simulink model "Dual_Sliding_Surface_Control_Try2"  (R2021b)
settings: Solver=VariableStepAuto  StartTime=tspan(1)  StopTime=tspan(2)  MinStep=1e-4  RelTol=1e-7
undefined symbols (not defined in the file): lambda_beta_num, lambda_gamma_num, lambda_x_num, lambda_y_num, r_sim, x_0
libraries: simulink_extras x2
settings Model: Creator=domin  LastModifiedBy=domin
settings SolverCC: AlgebraicLoopSolver=TrustRegion
settings DebuggingCC: SFMachineParentedDataDiag=warning

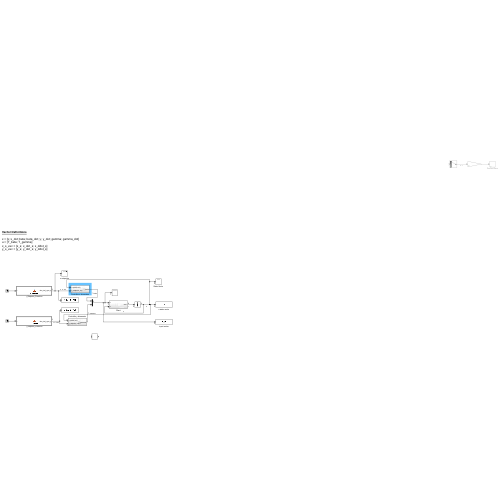
[thumbnail: Simulink's stored preview of the top-level diagram]
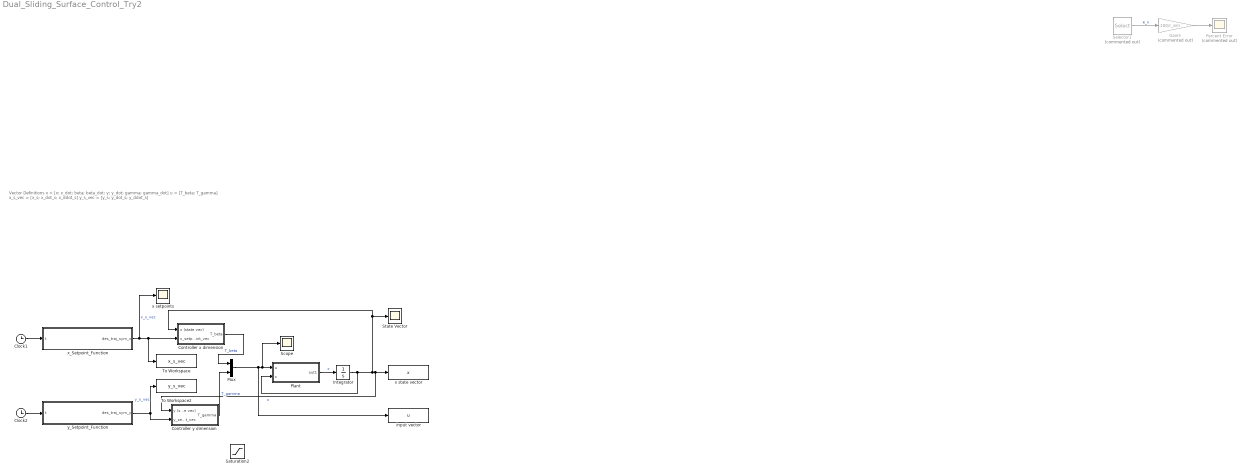
== system Dual_Sliding_Surface_Control_Try2 ==
  note: Vector Definitions
      |
      | x = [x; x_dot; beta; beta_dot; y; y_dot; gamma; gamma_dot]
      | u = [T_beta; T_gamma]
      | x_s_vec = [x_s; x_dot_s; x_ddot_s]
      | y_s_vec = [y_s; y_dot_s; y_ddot_s]
  Clock1 : Clock
  Clock2 : Clock
  Controller x dimension : Subsystem
  Controller y dimension : Subsystem
  Gain5 : Gain  Commented=on  Gain=100/r_sim
  Integrator : Integrator  InitialCondition=x_0
  Mux : Mux  Inputs=2
  Percent Error : Scope  Commented=on
  Plant : Subsystem
  Saturation2 : Saturate  UpperLimit=75/1000  LowerLimit=-75/1000  ZeroCross=off
  Scope : Scope
  Selector1 : Selector  Commented=on  InputPortWidth=5  IndexOptions=Index vector (dialog)  Indices=[1]  OutputSizes=1
  State Vector : Scope
  To Workspace : ToWorkspace  VariableName=x_s_vec  SampleTime=-1
  To Workspace2 : ToWorkspace  VariableName=y_s_vec  SampleTime=-1
  input vector : ToWorkspace  VariableName=u  SampleTime=-1
  x setpoints : Scope
  x state vector : ToWorkspace  VariableName=x  SampleTime=-1
  x_Setpoint_Function : MATLAB Function  TreatAsAtomicUnit=on
  y_Setpoint_Function : MATLAB Function  TreatAsAtomicUnit=on
  wires:
  x_Setpoint_Function/1(des_traj_sym_x) -> x setpoints/1, To Workspace/1, Controller x dimension/2(x_setpoint_vec)  "x_s_vec"
  Integrator/1 -> Plant/2(x), Controller y dimension/1(y (state vec)), x state vector/1, Controller x dimension/1(x (state vec)), State Vector/1  "x"
  Plant/1(out1) -> Integrator/1  "x"
  Clock1/1 -> x_Setpoint_Function/1(t)
  Gain5/1 -> Percent Error/1
  Selector1/1 -> Gain5/1  "e_x"
  Clock2/1 -> y_Setpoint_Function/1(t)
  Controller x dimension/1(T_beta) -> Mux/1  "T_beta"
  Controller y dimension/1(T_gamma) -> Mux/2  "T_gamma"
  y_Setpoint_Function/1(des_traj_sym_y) -> Controller y dimension/2(y_setpoint_vec), To Workspace2/1  "y_s_vec"
  Mux/1 -> Scope/1, Plant/1(u), input vector/1

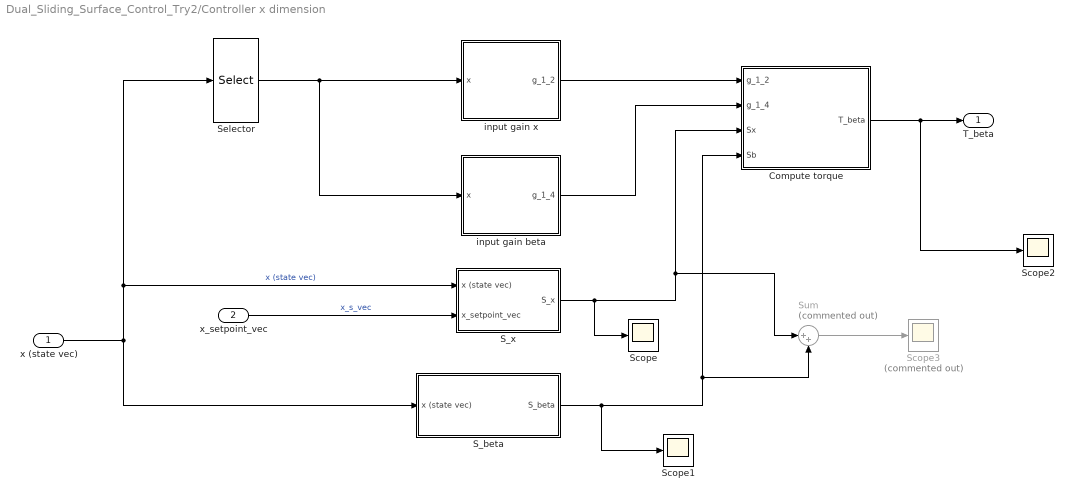
== system Dual_Sliding_Surface_Control_Try2/Controller x dimension ==
  x (state vec) : Inport
  x_setpoint_vec : Inport  Port=2
  Compute torque : MATLAB Function  TreatAsAtomicUnit=on
  S_beta : Subsystem
  S_x : Subsystem
  Scope : Scope
  Scope1 : Scope
  Scope2 : Scope
  Scope3 : Scope  Commented=on
  Selector : Selector  InputPortWidth=8  IndexOptions=Index vector (dialog)  Indices=[1]  OutputSizes=1
  Sum : Sum  Commented=on  Inputs=|++
  input gain beta : MATLAB Function  TreatAsAtomicUnit=on
  input gain x : MATLAB Function  TreatAsAtomicUnit=on
  T_beta : Outport
  wires:
  x (state vec)/1 -> Selector/1, S_x/1(x (state vec)), S_beta/1(x (state vec))  "x (state vec)"
  Selector/1 -> input gain beta/1(x), input gain x/1(x)
  x_setpoint_vec/1 -> S_x/2(x_setpoint_vec)  "x_s_vec"
  input gain x/1(g_1_2) -> Compute torque/1(g_1_2)
  input gain beta/1(g_1_4) -> Compute torque/2(g_1_4)
  S_x/1(S_x) -> Scope/1, Sum/1, Compute torque/3(Sx)
  S_beta/1(S_beta) -> Scope1/1, Sum/2, Compute torque/4(Sb)
  Compute torque/1(T_beta) -> T_beta/1, Scope2/1
  Sum/1 -> Scope3/1

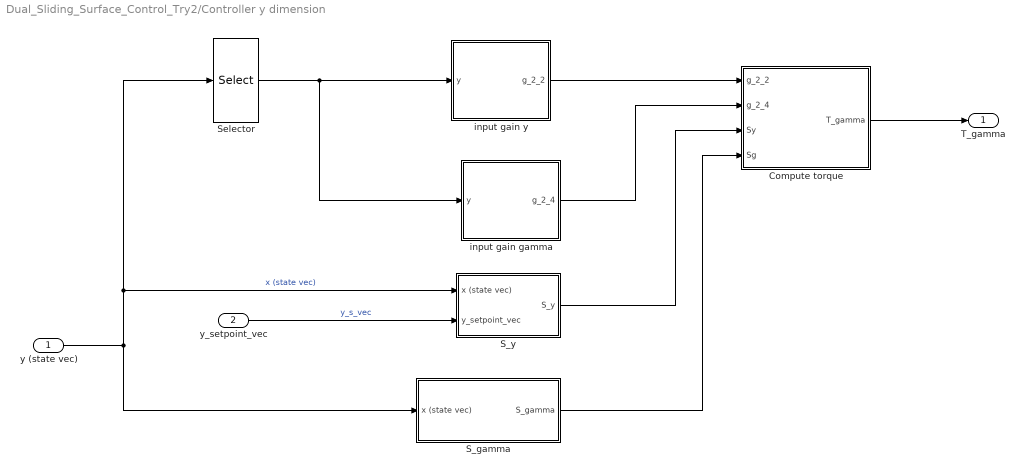
== system Dual_Sliding_Surface_Control_Try2/Controller y dimension ==
  y (state vec) : Inport
  y_setpoint_vec : Inport  Port=2
  Compute torque : MATLAB Function  TreatAsAtomicUnit=on
  S_gamma : Subsystem
  S_y : Subsystem
  Selector : Selector  InputPortWidth=8  IndexOptions=Index vector (dialog)  Indices=[5]  OutputSizes=1
  input gain gamma : MATLAB Function  TreatAsAtomicUnit=on
  input gain y : MATLAB Function  TreatAsAtomicUnit=on
  T_gamma : Outport
  wires:
  S_y/1(S_y) -> Compute torque/3(Sy)
  Compute torque/1(T_gamma) -> T_gamma/1
  input gain y/1(g_2_2) -> Compute torque/1(g_2_2)
  Selector/1 -> input gain gamma/1(y), input gain y/1(y)
  y_setpoint_vec/1 -> S_y/2(y_setpoint_vec)  "y_s_vec"
  input gain gamma/1(g_2_4) -> Compute torque/2(g_2_4)
  y (state vec)/1 -> Selector/1, S_y/1(x (state vec)), S_gamma/1(x (state vec))  "x (state vec)"
  S_gamma/1(S_gamma) -> Compute torque/4(Sg)

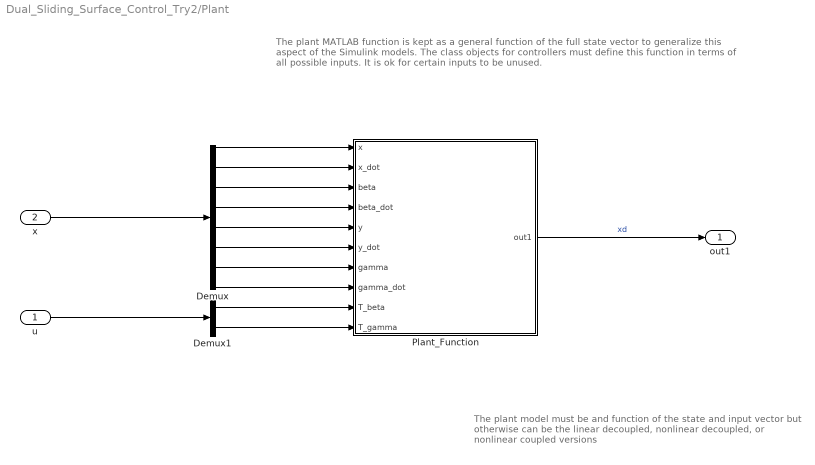
== system Dual_Sliding_Surface_Control_Try2/Plant ==
  note: The plant MATLAB function is kept as a general function of the full state vector
      | to generalize this aspect of the Simulink models. The class objects for controllers must define this function in terms of all possible inputs. It is ok for certain inputs to be unused.
  note: The plant model must be and function of the state and input vector
      |  but otherwise can be the linear decoupled, nonlinear decoupled,
      | or nonlinear coupled versions
  u : Inport
  x : Inport  Port=2
  Demux : Demux  Outputs=8
  Demux1 : Demux  Outputs=2
  Plant_Function : MATLAB Function  TreatAsAtomicUnit=on
  out1 : Outport
  wires:
  Demux1/1 -> Plant_Function/9(T_beta)
  Demux1/2 -> Plant_Function/10(T_gamma)
  Demux/5 -> Plant_Function/5(y)
  Demux/8 -> Plant_Function/8(gamma_dot)
  Demux/7 -> Plant_Function/7(gamma)
  Demux/1 -> Plant_Function/1(x)
  Demux/3 -> Plant_Function/3(beta)
  Demux/4 -> Plant_Function/4(beta_dot)
  Demux/2 -> Plant_Function/2(x_dot)
  Demux/6 -> Plant_Function/6(y_dot)
  x/1 -> Demux/1
  Plant_Function/1(out1) -> out1/1  "xd"
  u/1 -> Demux1/1

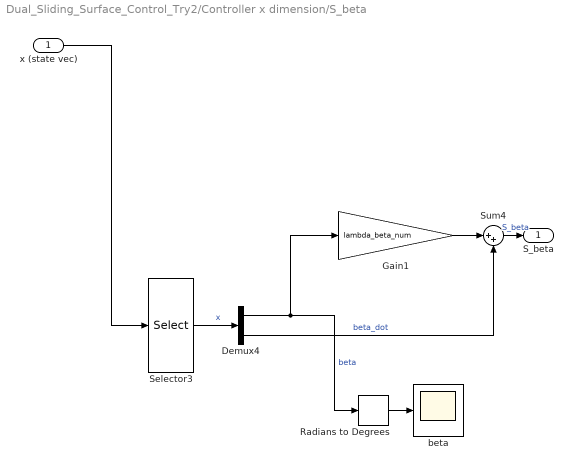
== system Dual_Sliding_Surface_Control_Try2/Controller x dimension/S_beta ==
  x (state vec) : Inport
  Demux4 : Demux  Outputs=2
  Gain1 : Gain  Gain=lambda_beta_num
  Radians to Degrees : simulink_extras/Transformations/Radians to Degrees
  Selector3 : Selector  InputPortWidth=8  IndexOptions=Index vector (dialog)  Indices=[3 4]  OutputSizes=1
  Sum4 : Sum  Inputs=|++
  beta : Scope
  S_beta : Outport
  wires:
  x (state vec)/1 -> Selector3/1
  Sum4/1 -> S_beta/1  "S_beta"
  Demux4/1 -> Gain1/1, Radians to Degrees/1  "beta"
  Gain1/1 -> Sum4/1
  Demux4/2 -> Sum4/2  "beta_dot"
  Radians to Degrees/1 -> beta/1
  Selector3/1 -> Demux4/1  "x"

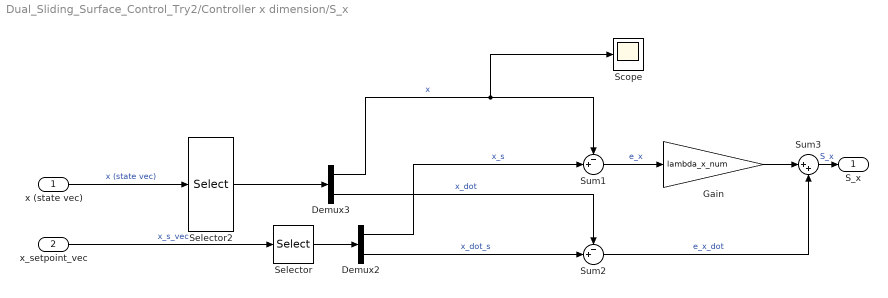
== system Dual_Sliding_Surface_Control_Try2/Controller x dimension/S_x ==
  x (state vec) : Inport
  x_setpoint_vec : Inport  Port=2
  Demux2 : Demux  Outputs=2
  Demux3 : Demux  Outputs=2
  Gain : Gain  Gain=lambda_x_num
  Scope : Scope
  Selector : Selector  InputPortWidth=3  IndexOptions=Index vector (dialog)  Indices=[1 2]  OutputSizes=1
  Selector2 : Selector  InputPortWidth=8  IndexOptions=Index vector (dialog)  Indices=[1 2]  OutputSizes=1
  Sum1 : Sum  Inputs=-+|
  Sum2 : Sum  Inputs=-+|
  Sum3 : Sum  Inputs=|++
  S_x : Outport
  wires:
  Gain/1 -> Sum3/1
  Sum1/1 -> Gain/1  "e_x"
  Sum2/1 -> Sum3/2  "e_x_dot"
  Demux3/1 -> Scope/1, Sum1/1  "x"
  Demux3/2 -> Sum2/1  "x_dot"
  Sum3/1 -> S_x/1  "S_x"
  x_setpoint_vec/1 -> Selector/1  "x_s_vec"
  x (state vec)/1 -> Selector2/1  "x (state vec)"
  Demux2/2 -> Sum2/2  "x_dot_s"
  Demux2/1 -> Sum1/2  "x_s"
  Selector2/1 -> Demux3/1
  Selector/1 -> Demux2/1

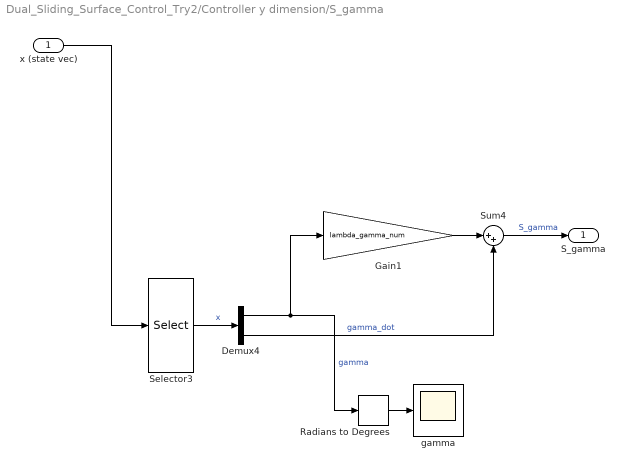
== system Dual_Sliding_Surface_Control_Try2/Controller y dimension/S_gamma ==
  x (state vec) : Inport
  Demux4 : Demux  Outputs=2
  Gain1 : Gain  Gain=lambda_gamma_num
  Radians to Degrees : simulink_extras/Transformations/Radians to Degrees
  Selector3 : Selector  InputPortWidth=8  IndexOptions=Index vector (dialog)  Indices=[7 8]  OutputSizes=1
  Sum4 : Sum  Inputs=|++
  gamma : Scope
  S_gamma : Outport
  wires:
  x (state vec)/1 -> Selector3/1
  Sum4/1 -> S_gamma/1  "S_gamma"
  Demux4/1 -> Gain1/1, Radians to Degrees/1  "gamma"
  Gain1/1 -> Sum4/1
  Demux4/2 -> Sum4/2  "gamma_dot"
  Radians to Degrees/1 -> gamma/1
  Selector3/1 -> Demux4/1  "x"

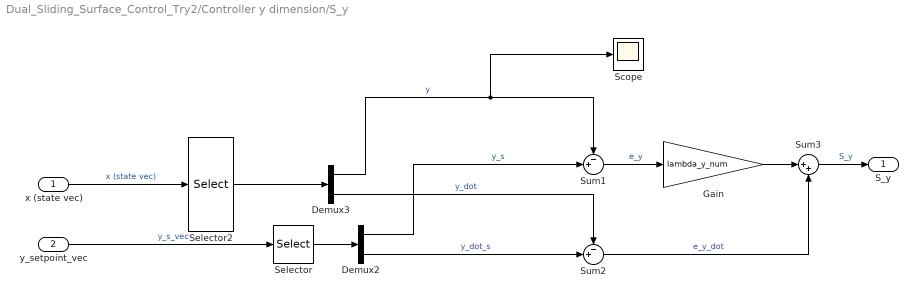
== system Dual_Sliding_Surface_Control_Try2/Controller y dimension/S_y ==
  x (state vec) : Inport
  y_setpoint_vec : Inport  Port=2
  Demux2 : Demux  Outputs=2
  Demux3 : Demux  Outputs=2
  Gain : Gain  Gain=lambda_y_num
  Scope : Scope
  Selector : Selector  InputPortWidth=3  IndexOptions=Index vector (dialog)  Indices=[1 2]  OutputSizes=1
  Selector2 : Selector  InputPortWidth=8  IndexOptions=Index vector (dialog)  Indices=[5 6]  OutputSizes=1
  Sum1 : Sum  Inputs=-+|
  Sum2 : Sum  Inputs=-+|
  Sum3 : Sum  Inputs=|++
  S_y : Outport
  wires:
  Gain/1 -> Sum3/1
  Sum1/1 -> Gain/1  "e_y"
  Sum2/1 -> Sum3/2  "e_y_dot"
  Demux3/1 -> Scope/1, Sum1/1  "y"
  Demux3/2 -> Sum2/1  "y_dot"
  Sum3/1 -> S_y/1  "S_y"
  y_setpoint_vec/1 -> Selector/1  "y_s_vec"
  x (state vec)/1 -> Selector2/1  "x (state vec)"
  Demux2/2 -> Sum2/2  "y_dot_s"
  Demux2/1 -> Sum1/2  "y_s"
  Selector2/1 -> Demux3/1
  Selector/1 -> Demux2/1

== matlab function Dual_Sliding_Surface_Control_Try2/Plant/Plant_Function ==
  data: x input; out1 output size=8; x_dot input; beta input; beta_dot input; y input; y_dot input; gamma input; gamma_dot input; T_beta input; T_gamma input
function out1 = xdot(x,x_dot,beta,beta_dot,y,y_dot,gamma,gamma_dot,T_beta,T_gamma)
%#codegen

%    This function was generated by the Symbolic Math Toolbox version 9.0.
%    14-Nov-2021 19:23:17

t2 = cos(beta);
t3 = cos(gamma);
t4 = sin(beta);
t5 = sin(gamma);
t6 = beta_dot.^2;
t7 = gamma_dot.^2;
t8 = x.^2;
t9 = y.^2;
t10 = t8.*(2.1e+1./1.0e+2);
t11 = t9.*(2.1e+1./1.0e+2);
t12 = t10+1.82492e-2;
t13 = t11+1.82492e-2;
t14 = 1.0./t12;
t15 = 1.0./t13;
mt1 = [x_dot,T_beta.*t14.*(-3.235e-1)+t14.*(t4.*7.3199277e-2+t4.*t8.*1.4715-t2.*x.*9.520605e-2+t6.*x.*1.34836525e-2+t6.*x.^3.*(3.0./2.0e+1)+beta_dot.*x.*x_dot.*1.941e-2),beta_dot,T_beta.*t14.*7.0+t14.*(t4.*1.183086+t2.*x.*2.0601-t6.*x.*9.705e-3-beta_dot.*x.*x_dot.*(2.1e+1./5.0e+1)),y_dot];
mt2 = [T_gamma.*t15.*3.235e-1-t15.*(t5.*7.3199277e-2+t5.*t9.*1.4715+t3.*y.*9.520605e-2-t7.*y.*1.34836525e-2-t7.*y.^3.*(3.0./2.0e+1)+gamma_dot.*y.*y_dot.*1.941e-2),gamma_dot,T_gamma.*t15.*7.0+t15.*(t5.*1.183086-t3.*y.*2.0601+t7.*y.*9.705e-3-gamma_dot.*y.*y_dot.*(2.1e+1./5.0e+1))];
out1 = reshape([mt1,mt2],8,1);

== matlab function Dual_Sliding_Surface_Control_Try2/x_Setpoint_Function ==
  data: t input; des_traj_sym_x output
function des_traj_sym_x = x_setpoint(t)
%#codegen

%    This function was generated by the Symbolic Math Toolbox version 9.0.
%    14-Nov-2021 19:23:17

t2 = t.*pi.*2.0;
t5 = t./3.0;
t3 = cos(t2);
t4 = sin(t2);
t6 = -t5;
t7 = exp(t6);
t8 = t7-1.0;
des_traj_sym_x = [t4.*t8.*(-1.0./5.0);(t4.*t7)./1.5e+1-t3.*t8.*pi.*(2.0./5.0);t4.*t7.*(-1.0./4.5e+1)+t3.*t7.*pi.*(4.0./1.5e+1)+t4.*t8.*pi.^2.*(4.0./5.0)];

== matlab function Dual_Sliding_Surface_Control_Try2/y_Setpoint_Function ==
  data: t input; des_traj_sym_y output
function des_traj_sym_y = y_setpoint(t)
%#codegen

%    This function was generated by the Symbolic Math Toolbox version 9.0.
%    14-Nov-2021 19:23:17

t2 = t.*pi.*2.0;
t5 = t./3.0;
t3 = cos(t2);
t4 = sin(t2);
t6 = -t5;
t7 = exp(t6);
t8 = t3.^2;
t9 = t4.^2;
t10 = t7-1.0;
des_traj_sym_y = [t3.*t4.*t10.*(-1.0./5.0);t8.*t10.*pi.*(-2.0./5.0)+t9.*t10.*pi.*(2.0./5.0)+(t3.*t4.*t7)./1.5e+1;t7.*t8.*pi.*(4.0./1.5e+1)-t7.*t9.*pi.*(4.0./1.5e+1)-(t3.*t4.*t7)./4.5e+1+t3.*t4.*t10.*pi.^2.*(1.6e+1./5.0)];

== matlab function Dual_Sliding_Surface_Control_Try2/Controller y dimension/Compute torque ==
  data: g_2_2 input; g_2_4 input; Tmax parameter; Sy input; T_gamma output; Sg input
function T_gamma = fcn(g_2_2, g_2_4, Tmax, Sy, Sg)

T_gamma= -Tmax*sign(Sg*g_2_4 - Sy*g_2_2);

== matlab function Dual_Sliding_Surface_Control_Try2/Controller x dimension/input gain x ==
  data: x input; g_1_2 output
function g_1_2 = g_1_2(x)
%#codegen

%    This function was generated by the Symbolic Math Toolbox version 9.0.
%    14-Nov-2021 21:51:26

g_1_2 = (-3.235e-1)./(x.^2.*(2.1e+1./1.0e+2)+1.82492e-2);

== matlab function Dual_Sliding_Surface_Control_Try2/Controller x dimension/input gain beta ==
  data: x input; g_1_4 output
function g_1_4 = g_1_4(x)
%#codegen

%    This function was generated by the Symbolic Math Toolbox version 9.0.
%    14-Nov-2021 21:51:26

g_1_4 = 7.0./(x.^2.*(2.1e+1./1.0e+2)+1.82492e-2);

== matlab function Dual_Sliding_Surface_Control_Try2/Controller x dimension/Compute torque ==
  data: g_1_2 input; g_1_4 input; Tmax parameter; Sx input; T_beta output; Sb input
function T_beta = fcn(g_1_2, g_1_4, Tmax, Sx, Sb)

T_beta = -Tmax*sign(Sb*g_1_4 - Sx*g_1_2);

% S = (Sb+Sx);
% T_beta = -Tmax*sign(S*(g_1_4-g_1_2));

== matlab function Dual_Sliding_Surface_Control_Try2/Controller y dimension/input gain gamma ==
  data: y input; g_2_4 output
function g_2_4 = g_2_4(y)
%#codegen

%    This function was generated by the Symbolic Math Toolbox version 9.0.
%    14-Nov-2021 21:51:26

g_2_4 = 7.0./(y.^2.*(2.1e+1./1.0e+2)+1.82492e-2);

== matlab function Dual_Sliding_Surface_Control_Try2/Controller y dimension/input gain y ==
  data: y input; g_2_2 output
function g_2_2 = g_2_2(y)
%#codegen

%    This function was generated by the Symbolic Math Toolbox version 9.0.
%    14-Nov-2021 21:51:26

g_2_2 = 3.235e-1./(y.^2.*(2.1e+1./1.0e+2)+1.82492e-2);
